simulink model "Tester"  (R2013b)
settings: Solver=ode3  StartTime=0.0  StopTime=SimEndTime  FixedStep=0.001  RelTol=1e-3
undefined symbols (not defined in the file or in its folder): DiscIntNeverNeededParam
settings Model: Creator=Sam  LastModifiedBy=Sam

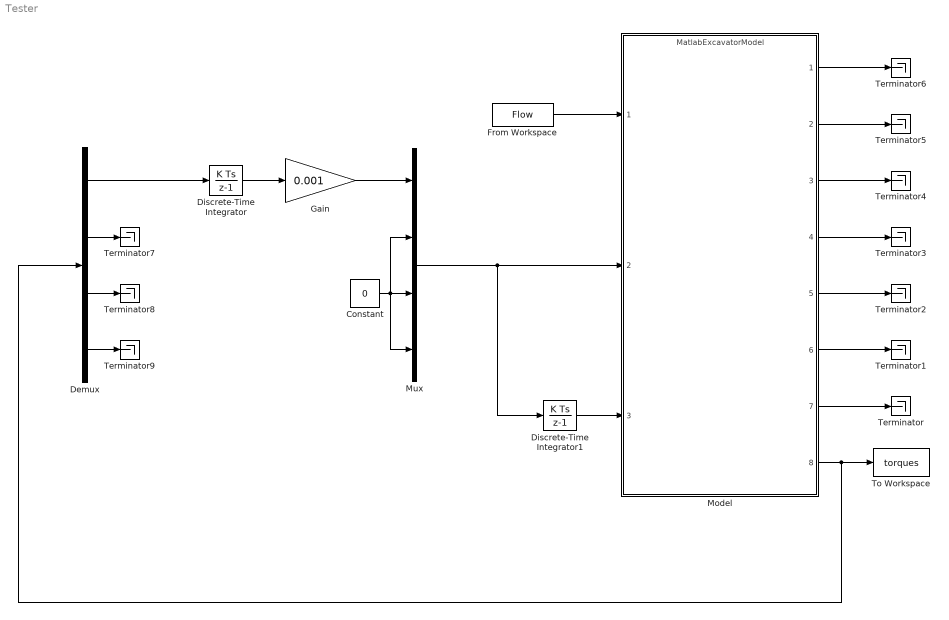
== system Tester ==
  Constant : Constant  Value=0
  Demux : Demux
  Discrete-Time Integrator : DiscreteIntegrator  SampleTime=-1  ICPrevOutput=DiscIntNeverNeededParam  ICPrevScaledInput=DiscIntNeverNeededParam
  Discrete-Time Integrator1 : DiscreteIntegrator  SampleTime=-1  ICPrevOutput=DiscIntNeverNeededParam  ICPrevScaledInput=DiscIntNeverNeededParam
  From Workspace : FromWorkspace  VariableName=Flow  SampleTime=0
  Gain : Gain  Gain=0.001
  Model : ModelReference  ModelNameDialog=MatlabExcavatorModel.slx  SimulationMode=Normal  Variant=on  OverrideUsingVariant=varObject  ModelReferenceVersion=1.227  CopyOfModelName=MatlabExcavatorModel.slx  DefaultDataLogging=on
  Mux : Mux
  Terminator{,1..9} (10 alike) : Terminator
  To Workspace : ToWorkspace  VariableName=torques  SampleTime=-1
  wires:
  From Workspace/1 -> Model/1
  Mux/1 -> Discrete-Time Integrator1/1, Model/2
  Model/7 -> Terminator/1
  Model/1 -> Terminator6/1
  Model/2 -> Terminator5/1
  Model/3 -> Terminator4/1
  Model/4 -> Terminator3/1
  Model/5 -> Terminator2/1
  Model/6 -> Terminator1/1
  Model/8 -> Demux/1, To Workspace/1
  Demux/2 -> Terminator7/1
  Demux/3 -> Terminator8/1
  Demux/4 -> Terminator9/1
  Constant/1 -> Mux/2, Mux/3, Mux/4
  Demux/1 -> Discrete-Time Integrator/1
  Gain/1 -> Mux/1
  Discrete-Time Integrator/1 -> Gain/1
  Discrete-Time Integrator1/1 -> Model/3
